simulink model "Estimations"  (R2023a)
settings: Solver=FixedStepAuto  StartTime=0.0  StopTime=150000  FixedStep=1  RelTol=1e-3
InitFcn:
  | load BatteryParameters.mat
values from neighbouring files (symbols this model uses):
  C1_LUT = [540 560 568 572 576 580 600 620 640 660 680 700 ... (105 elements, 21x5)]    [BatteryParameters.mat]
  Em_LUT = [3.147 3.292 3.392 3.477 3.518 3.561 3.602 3.638 3.677 3.719 3.763 3.799 ... (105 elements, 21x5)]    [BatteryParameters.mat]
  R1_LUT = [0.153117539 0.114898532 0.101253199 0.093222981 0.089962592 0.089117306 0.088090887 0.087366356 0.086883336 0.086038049 0.08477012 0.085313519 ... (105 elements, 21x5)]    [BatteryParameters.mat]
  SOC_LUT = [0 0.05 0.1 0.15 0.2 0.25 0.3 0.35 0.4 0.45 0.5 0.55 ... (21 elements, 21x1)]    [BatteryParameters.mat]
  Temperature_LUT = [263.15 273.15 298.15 318.15 333.15]    [BatteryParameters.mat]
  Ts = 1    [BatteryParameters.mat]
libraries: sharedTrackingLibrary x9
(part 1 of 2)
settings Model: Creator=The MathWorks, Inc.  LastModifiedBy=10661326
settings SolverCC: AlgebraicLoopSolver=TrustRegion
settings DataIOCC: ReturnWorkspaceOutputs=off
settings OptimizationCC: DefaultParameterBehavior=Inlined  EnhancedBackFolding=on  PassReuseOutputArgsAs=Individual arguments  ZeroExternalMemoryAtStartup=off  ZeroInternalMemoryAtStartup=off  OptimizeBlockOrder=speed  DifferentSizesBufferReuse=on  OptimizationCustomize=off  EfficientTunableParamExpr=on
settings DebuggingCC: ParameterTunabilityLossMsg=error  UnconnectedInputMsg=warning  UnconnectedOutputMsg=warning  UnconnectedLineMsg=warning  ArithmeticOperatorsInVariantConditions=warning
settings HardwareCC: ProdBitPerChar=16  ProdBitPerInt=16  ProdBitPerPointer=32  ProdBitPerSizeT=32  ProdBitPerPtrDiffT=32  ProdLargestAtomicInteger=Integer  ProdLargestAtomicFloat=None  ProdWordSize=16  ProdHWDeviceType=Texas Instruments->C2000
settings ModelReferenceCC: EnableRefExpFcnMdlSchedulingChecks=on
settings SFSimCC: SimUseLocalCustomCode=off  MATLABDynamicMemAlloc=off  CustomCodeUndefinedFunction=UseInterfaceOnly
settings RTWCC: Description=Embedded Coder  SystemTargetFile=ert.tlc  TemplateMakefile=ert_default_tmf  RTWUseLocalCustomCode=off  DLArmComputeVersion=19.05
settings CodeAppCC: ForceParamTrailComments=on  IgnoreCustomStorageClasses=off  OperatorAnnotations=on  SimulinkDataObjDesc=on  SFDataObjDesc=on  InsertBlockDesc=on
settings ERTTargetCC: TargetLangStandard=C99 (ISO)  GenerateSampleERTMain=on  InlinedParameterPlacement=NonHierarchical  ERTCustomFileTemplate=example_file_process.tlc
settings SimscapeCC: SimscapeNormalizeSystem=off

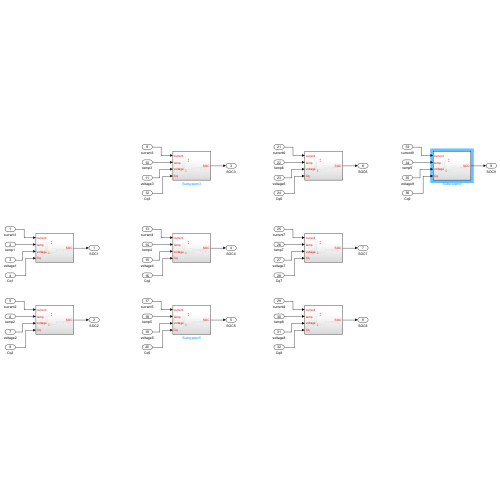
[thumbnail: Simulink's stored preview of the top-level diagram]
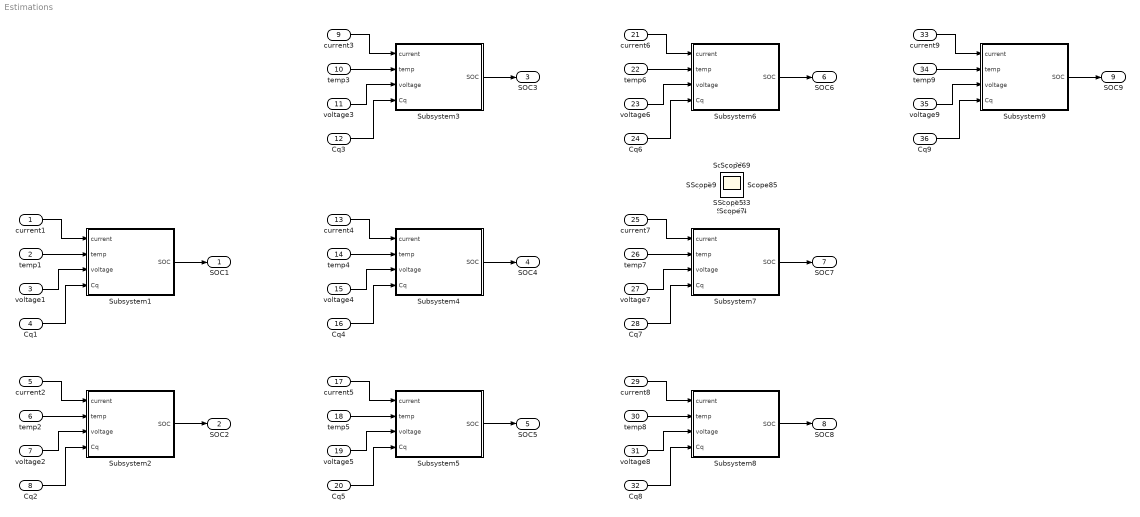
== system Estimations ==
  current1 : Inport
  temp1 : Inport  Port=2
  voltage1 : Inport  Port=3
  Cq1 : Inport  Port=4
  current2 : Inport  Port=5
  temp2 : Inport  Port=6
  voltage2 : Inport  Port=7
  Cq2 : Inport  Port=8
  current3 : Inport  Port=9
  temp3 : Inport  Port=10
  voltage3 : Inport  Port=11
  Cq3 : Inport  Port=12
  current4 : Inport  Port=13
  temp4 : Inport  Port=14
  voltage4 : Inport  Port=15
  Cq4 : Inport  Port=16
  current5 : Inport  Port=17
  temp5 : Inport  Port=18
  voltage5 : Inport  Port=19
  Cq5 : Inport  Port=20
  current6 : Inport  Port=21
  temp6 : Inport  Port=22
  voltage6 : Inport  Port=23
  Cq6 : Inport  Port=24
  current7 : Inport  Port=25
  temp7 : Inport  Port=26
  voltage7 : Inport  Port=27
  Cq7 : Inport  Port=28
  current8 : Inport  Port=29
  temp8 : Inport  Port=30
  voltage8 : Inport  Port=31
  Cq8 : Inport  Port=32
  current9 : Inport  Port=33
  temp9 : Inport  Port=34
  voltage9 : Inport  Port=35
  Cq9 : Inport  Port=36
  Subsystem1 : Subsystem
  Subsystem2 : Subsystem
  Subsystem3 : Subsystem
  Subsystem4 : Subsystem
  Subsystem5 : Subsystem
  Subsystem6 : Subsystem
  Subsystem7 : Subsystem
  Subsystem8 : Subsystem
  Subsystem9 : Subsystem
  SOC1 : Outport
  SOC2 : Outport  Port=2
  SOC3 : Outport  Port=3
  SOC4 : Outport  Port=4
  SOC5 : Outport  Port=5
  SOC6 : Outport  Port=6
  SOC7 : Outport  Port=7
  SOC8 : Outport  Port=8
  SOC9 : Outport  Port=9
  Scope{,1..11,13,17..18,20,22..35} (30 alike) : Scope
  wires:
  Subsystem1/1(SOC) -> SOC1/1
  Cq1/1 -> Subsystem1/4(Cq)
  current1/1 -> Subsystem1/1(current)
  temp1/1 -> Subsystem1/2(temp)
  voltage1/1 -> Subsystem1/3(voltage)
  voltage2/1 -> Subsystem2/3(voltage)
  temp2/1 -> Subsystem2/2(temp)
  current2/1 -> Subsystem2/1(current)
  Cq2/1 -> Subsystem2/4(Cq)
  Subsystem2/1(SOC) -> SOC2/1
  Subsystem5/1(SOC) -> SOC5/1
  Cq5/1 -> Subsystem5/4(Cq)
  current5/1 -> Subsystem5/1(current)
  temp5/1 -> Subsystem5/2(temp)
  voltage5/1 -> Subsystem5/3(voltage)
  voltage4/1 -> Subsystem4/3(voltage)
  temp4/1 -> Subsystem4/2(temp)
  current4/1 -> Subsystem4/1(current)
  Cq4/1 -> Subsystem4/4(Cq)
  Subsystem4/1(SOC) -> SOC4/1
  Subsystem3/1(SOC) -> SOC3/1
  Cq3/1 -> Subsystem3/4(Cq)
  current3/1 -> Subsystem3/1(current)
  temp3/1 -> Subsystem3/2(temp)
  voltage3/1 -> Subsystem3/3(voltage)
  voltage6/1 -> Subsystem6/3(voltage)
  temp6/1 -> Subsystem6/2(temp)
  current6/1 -> Subsystem6/1(current)
  Cq6/1 -> Subsystem6/4(Cq)
  Subsystem6/1(SOC) -> SOC6/1
  Subsystem7/1(SOC) -> SOC7/1
  Cq7/1 -> Subsystem7/4(Cq)
  current7/1 -> Subsystem7/1(current)
  temp7/1 -> Subsystem7/2(temp)
  voltage7/1 -> Subsystem7/3(voltage)
  voltage8/1 -> Subsystem8/3(voltage)
  temp8/1 -> Subsystem8/2(temp)
  current8/1 -> Subsystem8/1(current)
  Cq8/1 -> Subsystem8/4(Cq)
  Subsystem8/1(SOC) -> SOC8/1
  Subsystem9/1(SOC) -> SOC9/1
  Cq9/1 -> Subsystem9/4(Cq)
  current9/1 -> Subsystem9/1(current)
  temp9/1 -> Subsystem9/2(temp)
  voltage9/1 -> Subsystem9/3(voltage)

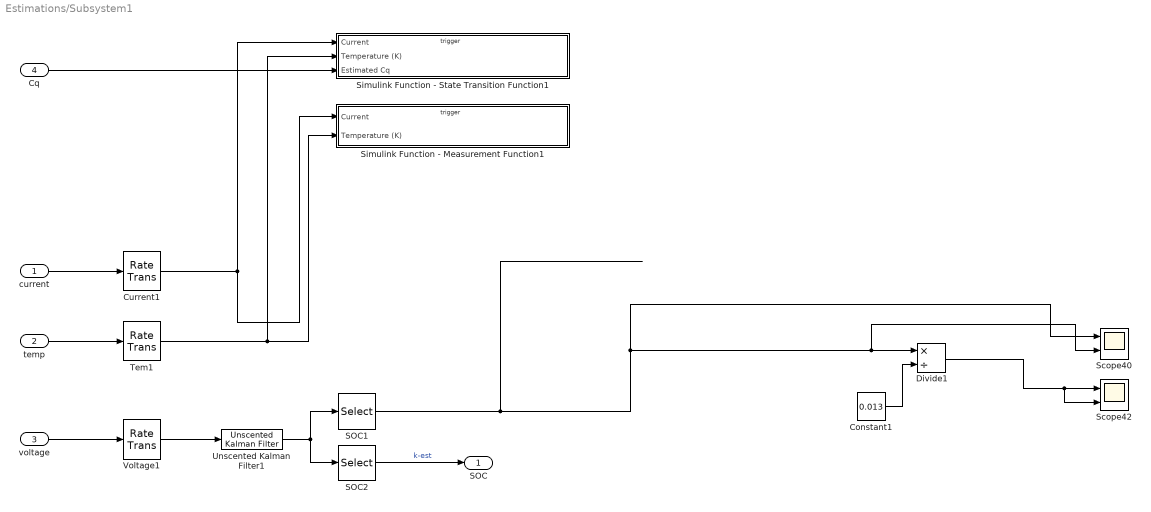
== system Estimations/Subsystem1 ==
  current : Inport
  temp : Inport  Port=2
  voltage : Inport  Port=3
  Cq : Inport  Port=4
  Constant1 : Constant  Value=0.013
  Current1 : RateTransition  OutPortSampleTime=Ts
  Divide1 : Product  Inputs=*/
  SOC1 : Selector  InputPortWidth=3  IndexOptions=Index vector (dialog)  Indices=3  OutputSizes=1
  SOC2 : Selector  InputPortWidth=3  IndexOptions=Index vector (dialog)  Indices=1  OutputSizes=1
  Scope40 : Scope  NumInputPorts=2
  Scope42 : Scope  NumInputPorts=2
  Simulink Function - Measurement Function1 : Subsystem  TreatAsAtomicUnit=on
  Simulink Function - State Transition Function1 : Subsystem  TreatAsAtomicUnit=on
  Tem1 : RateTransition  InitialCondition=300  OutPortSampleTime=Ts
  Unscented Kalman Filter1 : sharedTrackingLibrary/Unscented Kalman Filter  StateTransitionFcn=batteryStateFcn1  HasAdditiveProcessNoise=Additive  ProcessNoise=diag([2e-8, 3e-7, 2e-8])  HasTimeVaryingProcessNoise=off  HasStateTransitionFcnExtraArgument=0  InitialState=[0.5; 0; 0.01]  InitialStateCovariance=diag([0.01, 1,1])  Alpha=1  Beta=2  Kappa=0  MeasurementFcn1=batteryMeasurementFcn1  HasMeasurementEnablePort1=off  HasAdditiveMeasurementNoise1=Additive  MeasurementNoise1=1e-3  HasTimeVaryingMeasurementNoise1=off  HasMeasurementFcnExtraArgument1=0  HasMeasurementWrapping1=off  MeasurementFcn2=myMeasurementFcn  HasMeasurementEnablePort2=off  HasAdditiveMeasurementNoise2=Additive  MeasurementNoise2=1  HasTimeVaryingMeasurementNoise2=off  HasMeasurementFcnExtraArgument2=0  HasMeasurementWrapping2=off  MeasurementFcn3=myMeasurementFcn  HasMeasurementEnablePort3=off  HasAdditiveMeasurementNoise3=Additive  MeasurementNoise3=1  HasTimeVaryingMeasurementNoise3=off  HasMeasurementFcnExtraArgument3=0  HasMeasurementWrapping3=off  MeasurementFcn4=myMeasurementFcn  HasMeasurementEnablePort4=off  HasAdditiveMeasurementNoise4=Additive  MeasurementNoise4=1  HasTimeVaryingMeasurementNoise4=off  HasMeasurementFcnExtraArgument4=0  HasMeasurementWrapping4=off  MeasurementFcn5=myMeasurementFcn  HasMeasurementEnablePort5=off  HasAdditiveMeasurementNoise5=Additive  MeasurementNoise5=1  HasTimeVaryingMeasurementNoise5=off  HasMeasurementFcnExtraArgument5=0  HasMeasurementWrapping5=off  EnableMultirate=off  StateTransitionFcnSampleTime=-1  MeasurementFcn1SampleTime=-1  MeasurementFcn2SampleTime=-1  MeasurementFcn3SampleTime=-1  MeasurementFcn4SampleTime=-1  MeasurementFcn5SampleTime=-1  UseCurrentEstimator=on  OutputStateCovariance=off  DataType=double  SampleTime=Ts  NumberOfMeasurements=1
  Voltage1 : RateTransition  InitialCondition=4  OutPortSampleTime=Ts
  SOC : Outport
  wires:
  Cq/1 -> Simulink Function - State Transition Function1/3(Estimated Cq)
  voltage/1 -> Voltage1/1
  Tem1/1 -> Simulink Function - Measurement Function1/2(Temperature (K)), Simulink Function - State Transition Function1/2(Temperature (K))
  Current1/1 -> Simulink Function - State Transition Function1/1(Current), Simulink Function - Measurement Function1/1(Current)
  current/1 -> Current1/1
  temp/1 -> Tem1/1
  Divide1/1 -> Scope42/1, Scope42/2
  Unscented Kalman Filter1/1 -> SOC2/1, SOC1/1
  SOC2/1 -> SOC/1  "k-est"
  Voltage1/1 -> Unscented Kalman Filter1/1
  Constant1/1 -> Divide1/2
  SOC1/1 -> Scope40/1, Divide1/1, Scope40/2

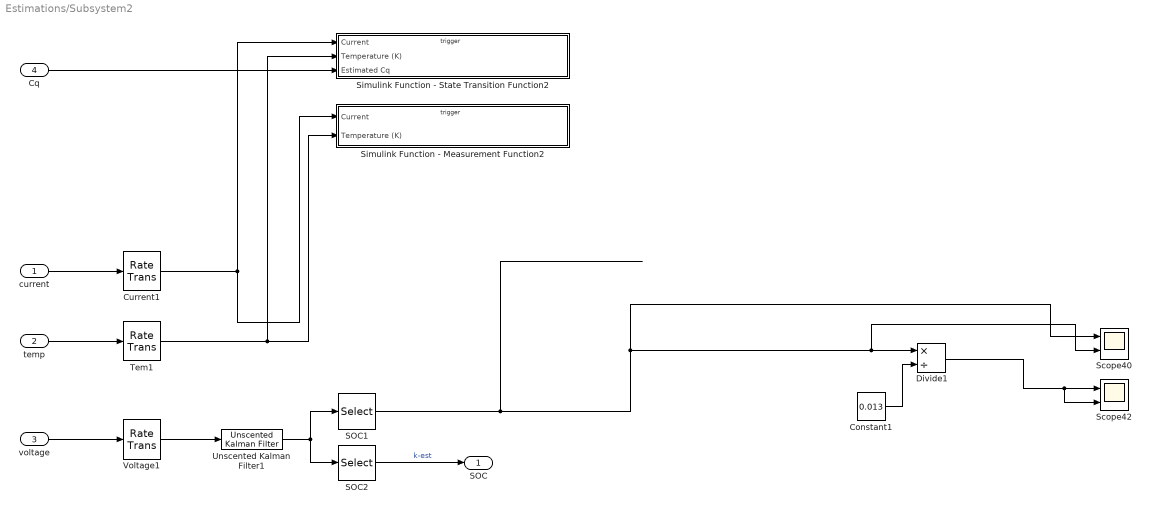
== system Estimations/Subsystem2 ==
  current : Inport
  temp : Inport  Port=2
  voltage : Inport  Port=3
  Cq : Inport  Port=4
  Constant1 : Constant  Value=0.013
  Current1 : RateTransition  OutPortSampleTime=Ts
  Divide1 : Product  Inputs=*/
  SOC1 : Selector  InputPortWidth=3  IndexOptions=Index vector (dialog)  Indices=3  OutputSizes=1
  SOC2 : Selector  InputPortWidth=3  IndexOptions=Index vector (dialog)  Indices=1  OutputSizes=1
  Scope40 : Scope  NumInputPorts=2
  Scope42 : Scope  NumInputPorts=2
  Simulink Function - Measurement Function2 : Subsystem  TreatAsAtomicUnit=on
  Simulink Function - State Transition Function2 : Subsystem  TreatAsAtomicUnit=on
  Tem1 : RateTransition  InitialCondition=300  OutPortSampleTime=Ts
  Unscented Kalman Filter1 : sharedTrackingLibrary/Unscented Kalman Filter  StateTransitionFcn=batteryStateFcn2  HasAdditiveProcessNoise=Additive  ProcessNoise=diag([2e-8, 3e-7, 2e-8])  HasTimeVaryingProcessNoise=off  HasStateTransitionFcnExtraArgument=0  InitialState=[0.5; 0; 0.01]  InitialStateCovariance=diag([0.01, 1,1])  Alpha=1  Beta=2  Kappa=0  MeasurementFcn1=batteryMeasurementFcn2  HasMeasurementEnablePort1=off  HasAdditiveMeasurementNoise1=Additive  MeasurementNoise1=1e-3  HasTimeVaryingMeasurementNoise1=off  HasMeasurementFcnExtraArgument1=0  HasMeasurementWrapping1=off  MeasurementFcn2=myMeasurementFcn  HasMeasurementEnablePort2=off  HasAdditiveMeasurementNoise2=Additive  MeasurementNoise2=1  HasTimeVaryingMeasurementNoise2=off  HasMeasurementFcnExtraArgument2=0  HasMeasurementWrapping2=off  MeasurementFcn3=myMeasurementFcn  HasMeasurementEnablePort3=off  HasAdditiveMeasurementNoise3=Additive  MeasurementNoise3=1  HasTimeVaryingMeasurementNoise3=off  HasMeasurementFcnExtraArgument3=0  HasMeasurementWrapping3=off  MeasurementFcn4=myMeasurementFcn  HasMeasurementEnablePort4=off  HasAdditiveMeasurementNoise4=Additive  MeasurementNoise4=1  HasTimeVaryingMeasurementNoise4=off  HasMeasurementFcnExtraArgument4=0  HasMeasurementWrapping4=off  MeasurementFcn5=myMeasurementFcn  HasMeasurementEnablePort5=off  HasAdditiveMeasurementNoise5=Additive  MeasurementNoise5=1  HasTimeVaryingMeasurementNoise5=off  HasMeasurementFcnExtraArgument5=0  HasMeasurementWrapping5=off  EnableMultirate=off  StateTransitionFcnSampleTime=-1  MeasurementFcn1SampleTime=-1  MeasurementFcn2SampleTime=-1  MeasurementFcn3SampleTime=-1  MeasurementFcn4SampleTime=-1  MeasurementFcn5SampleTime=-1  UseCurrentEstimator=on  OutputStateCovariance=off  DataType=double  SampleTime=Ts  NumberOfMeasurements=1
  Voltage1 : RateTransition  InitialCondition=4  OutPortSampleTime=Ts
  SOC : Outport
  wires:
  SOC1/1 -> Scope40/2, Divide1/1, Scope40/1
  Constant1/1 -> Divide1/2
  Voltage1/1 -> Unscented Kalman Filter1/1
  SOC2/1 -> SOC/1  "k-est"
  Unscented Kalman Filter1/1 -> SOC1/1, SOC2/1
  Divide1/1 -> Scope42/2, Scope42/1
  temp/1 -> Tem1/1
  current/1 -> Current1/1
  Current1/1 -> Simulink Function - Measurement Function2/1(Current), Simulink Function - State Transition Function2/1(Current)
  Tem1/1 -> Simulink Function - State Transition Function2/2(Temperature (K)), Simulink Function - Measurement Function2/2(Temperature (K))
  voltage/1 -> Voltage1/1
  Cq/1 -> Simulink Function - State Transition Function2/3(Estimated Cq)

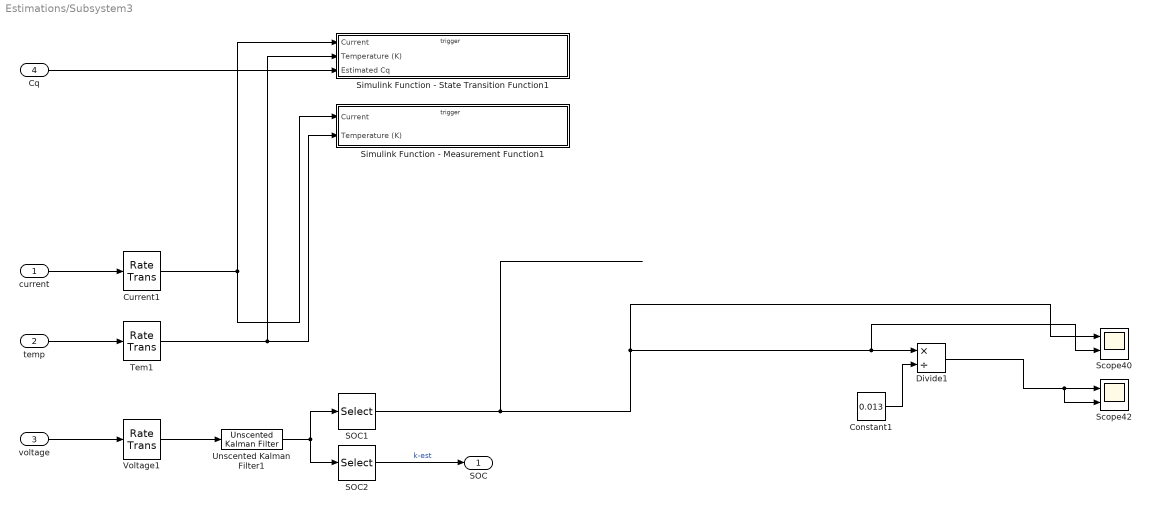
== system Estimations/Subsystem3 ==
  current : Inport
  temp : Inport  Port=2
  voltage : Inport  Port=3
  Cq : Inport  Port=4
  Constant1 : Constant  Value=0.013
  Current1 : RateTransition  OutPortSampleTime=Ts
  Divide1 : Product  Inputs=*/
  SOC1 : Selector  InputPortWidth=3  IndexOptions=Index vector (dialog)  Indices=3  OutputSizes=1
  SOC2 : Selector  InputPortWidth=3  IndexOptions=Index vector (dialog)  Indices=1  OutputSizes=1
  Scope40 : Scope  NumInputPorts=2
  Scope42 : Scope  NumInputPorts=2
  Simulink Function - Measurement Function1 : Subsystem  TreatAsAtomicUnit=on
  Simulink Function - State Transition Function1 : Subsystem  TreatAsAtomicUnit=on
  Tem1 : RateTransition  InitialCondition=300  OutPortSampleTime=Ts
  Unscented Kalman Filter1 : sharedTrackingLibrary/Unscented Kalman Filter  StateTransitionFcn=batteryStateFcn3  HasAdditiveProcessNoise=Additive  ProcessNoise=diag([2e-8, 3e-7, 2e-8])  HasTimeVaryingProcessNoise=off  HasStateTransitionFcnExtraArgument=0  InitialState=[0.5; 0; 0.01]  InitialStateCovariance=diag([0.01, 1,1])  Alpha=1  Beta=2  Kappa=0  MeasurementFcn1=batteryMeasurementFcn3  HasMeasurementEnablePort1=off  HasAdditiveMeasurementNoise1=Additive  MeasurementNoise1=1e-3  HasTimeVaryingMeasurementNoise1=off  HasMeasurementFcnExtraArgument1=0  HasMeasurementWrapping1=off  MeasurementFcn2=myMeasurementFcn  HasMeasurementEnablePort2=off  HasAdditiveMeasurementNoise2=Additive  MeasurementNoise2=1  HasTimeVaryingMeasurementNoise2=off  HasMeasurementFcnExtraArgument2=0  HasMeasurementWrapping2=off  MeasurementFcn3=myMeasurementFcn  HasMeasurementEnablePort3=off  HasAdditiveMeasurementNoise3=Additive  MeasurementNoise3=1  HasTimeVaryingMeasurementNoise3=off  HasMeasurementFcnExtraArgument3=0  HasMeasurementWrapping3=off  MeasurementFcn4=myMeasurementFcn  HasMeasurementEnablePort4=off  HasAdditiveMeasurementNoise4=Additive  MeasurementNoise4=1  HasTimeVaryingMeasurementNoise4=off  HasMeasurementFcnExtraArgument4=0  HasMeasurementWrapping4=off  MeasurementFcn5=myMeasurementFcn  HasMeasurementEnablePort5=off  HasAdditiveMeasurementNoise5=Additive  MeasurementNoise5=1  HasTimeVaryingMeasurementNoise5=off  HasMeasurementFcnExtraArgument5=0  HasMeasurementWrapping5=off  EnableMultirate=off  StateTransitionFcnSampleTime=-1  MeasurementFcn1SampleTime=-1  MeasurementFcn2SampleTime=-1  MeasurementFcn3SampleTime=-1  MeasurementFcn4SampleTime=-1  MeasurementFcn5SampleTime=-1  UseCurrentEstimator=on  OutputStateCovariance=off  DataType=double  SampleTime=Ts  NumberOfMeasurements=1
  Voltage1 : RateTransition  InitialCondition=4  OutPortSampleTime=Ts
  SOC : Outport
  wires:
  Cq/1 -> Simulink Function - State Transition Function1/3(Estimated Cq)
  voltage/1 -> Voltage1/1
  Tem1/1 -> Simulink Function - Measurement Function1/2(Temperature (K)), Simulink Function - State Transition Function1/2(Temperature (K))
  Current1/1 -> Simulink Function - State Transition Function1/1(Current), Simulink Function - Measurement Function1/1(Current)
  current/1 -> Current1/1
  temp/1 -> Tem1/1
  Divide1/1 -> Scope42/1, Scope42/2
  Unscented Kalman Filter1/1 -> SOC2/1, SOC1/1
  SOC2/1 -> SOC/1  "k-est"
  Voltage1/1 -> Unscented Kalman Filter1/1
  Constant1/1 -> Divide1/2
  SOC1/1 -> Scope40/1, Divide1/1, Scope40/2

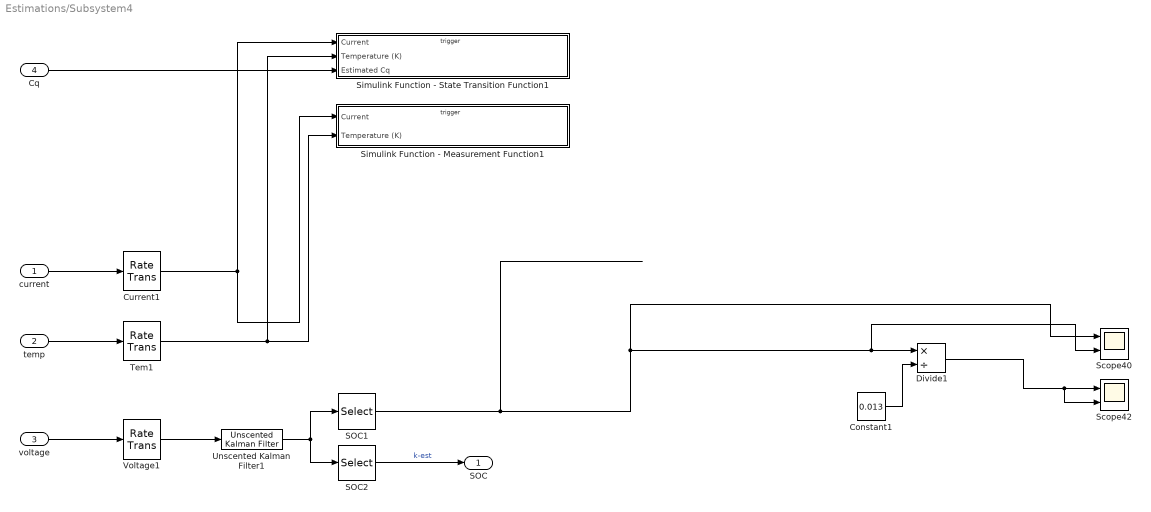
== system Estimations/Subsystem4 ==
  current : Inport
  temp : Inport  Port=2
  voltage : Inport  Port=3
  Cq : Inport  Port=4
  Constant1 : Constant  Value=0.013
  Current1 : RateTransition  OutPortSampleTime=Ts
  Divide1 : Product  Inputs=*/
  SOC1 : Selector  InputPortWidth=3  IndexOptions=Index vector (dialog)  Indices=3  OutputSizes=1
  SOC2 : Selector  InputPortWidth=3  IndexOptions=Index vector (dialog)  Indices=1  OutputSizes=1
  Scope40 : Scope  NumInputPorts=2
  Scope42 : Scope  NumInputPorts=2
  Simulink Function - Measurement Function1 : Subsystem  TreatAsAtomicUnit=on
  Simulink Function - State Transition Function1 : Subsystem  TreatAsAtomicUnit=on
  Tem1 : RateTransition  InitialCondition=300  OutPortSampleTime=Ts
  Unscented Kalman Filter1 : sharedTrackingLibrary/Unscented Kalman Filter  StateTransitionFcn=batteryStateFcn4  HasAdditiveProcessNoise=Additive  ProcessNoise=diag([2e-8, 3e-7, 2e-8])  HasTimeVaryingProcessNoise=off  HasStateTransitionFcnExtraArgument=0  InitialState=[0.5; 0; 0.01]  InitialStateCovariance=diag([0.01, 1,1])  Alpha=1  Beta=2  Kappa=0  MeasurementFcn1=batteryMeasurementFcn4  HasMeasurementEnablePort1=off  HasAdditiveMeasurementNoise1=Additive  MeasurementNoise1=1e-3  HasTimeVaryingMeasurementNoise1=off  HasMeasurementFcnExtraArgument1=0  HasMeasurementWrapping1=off  MeasurementFcn2=myMeasurementFcn  HasMeasurementEnablePort2=off  HasAdditiveMeasurementNoise2=Additive  MeasurementNoise2=1  HasTimeVaryingMeasurementNoise2=off  HasMeasurementFcnExtraArgument2=0  HasMeasurementWrapping2=off  MeasurementFcn3=myMeasurementFcn  HasMeasurementEnablePort3=off  HasAdditiveMeasurementNoise3=Additive  MeasurementNoise3=1  HasTimeVaryingMeasurementNoise3=off  HasMeasurementFcnExtraArgument3=0  HasMeasurementWrapping3=off  MeasurementFcn4=myMeasurementFcn  HasMeasurementEnablePort4=off  HasAdditiveMeasurementNoise4=Additive  MeasurementNoise4=1  HasTimeVaryingMeasurementNoise4=off  HasMeasurementFcnExtraArgument4=0  HasMeasurementWrapping4=off  MeasurementFcn5=myMeasurementFcn  HasMeasurementEnablePort5=off  HasAdditiveMeasurementNoise5=Additive  MeasurementNoise5=1  HasTimeVaryingMeasurementNoise5=off  HasMeasurementFcnExtraArgument5=0  HasMeasurementWrapping5=off  EnableMultirate=off  StateTransitionFcnSampleTime=-1  MeasurementFcn1SampleTime=-1  MeasurementFcn2SampleTime=-1  MeasurementFcn3SampleTime=-1  MeasurementFcn4SampleTime=-1  MeasurementFcn5SampleTime=-1  UseCurrentEstimator=on  OutputStateCovariance=off  DataType=double  SampleTime=Ts  NumberOfMeasurements=1
  Voltage1 : RateTransition  InitialCondition=4  OutPortSampleTime=Ts
  SOC : Outport
  wires:
  SOC1/1 -> Scope40/2, Divide1/1, Scope40/1
  Constant1/1 -> Divide1/2
  Voltage1/1 -> Unscented Kalman Filter1/1
  SOC2/1 -> SOC/1  "k-est"
  Unscented Kalman Filter1/1 -> SOC1/1, SOC2/1
  Divide1/1 -> Scope42/2, Scope42/1
  temp/1 -> Tem1/1
  current/1 -> Current1/1
  Current1/1 -> Simulink Function - Measurement Function1/1(Current), Simulink Function - State Transition Function1/1(Current)
  Tem1/1 -> Simulink Function - State Transition Function1/2(Temperature (K)), Simulink Function - Measurement Function1/2(Temperature (K))
  voltage/1 -> Voltage1/1
  Cq/1 -> Simulink Function - State Transition Function1/3(Estimated Cq)

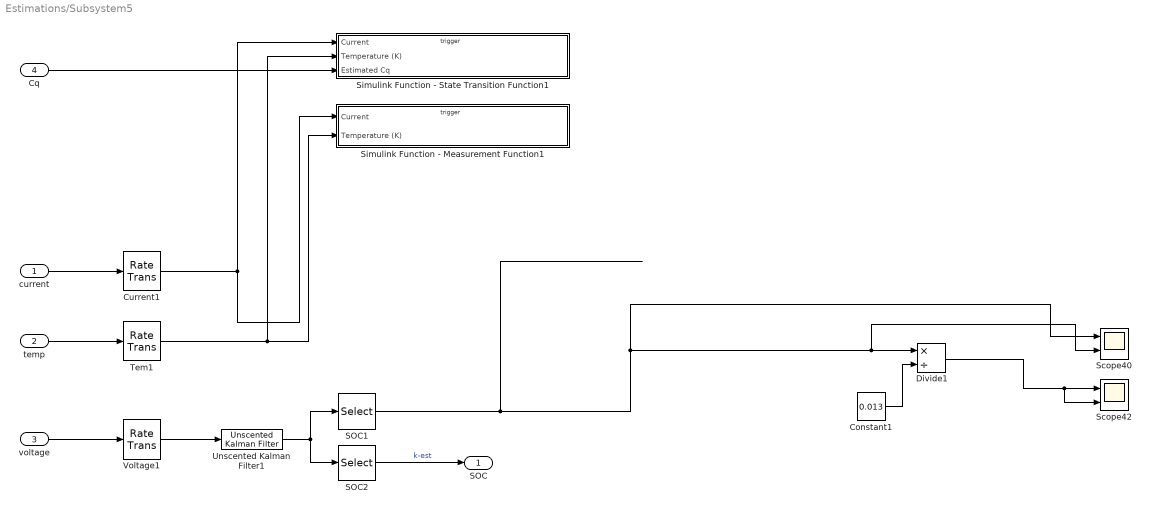
== system Estimations/Subsystem5 ==
  current : Inport
  temp : Inport  Port=2
  voltage : Inport  Port=3
  Cq : Inport  Port=4
  Constant1 : Constant  Value=0.013
  Current1 : RateTransition  OutPortSampleTime=Ts
  Divide1 : Product  Inputs=*/
  SOC1 : Selector  InputPortWidth=3  IndexOptions=Index vector (dialog)  Indices=3  OutputSizes=1
  SOC2 : Selector  InputPortWidth=3  IndexOptions=Index vector (dialog)  Indices=1  OutputSizes=1
  Scope40 : Scope  NumInputPorts=2
  Scope42 : Scope  NumInputPorts=2
  Simulink Function - Measurement Function1 : Subsystem  TreatAsAtomicUnit=on
  Simulink Function - State Transition Function1 : Subsystem  TreatAsAtomicUnit=on
  Tem1 : RateTransition  InitialCondition=300  OutPortSampleTime=Ts
  Unscented Kalman Filter1 : sharedTrackingLibrary/Unscented Kalman Filter  StateTransitionFcn=batteryStateFcn5  HasAdditiveProcessNoise=Additive  ProcessNoise=diag([2e-8, 3e-7, 2e-8])  HasTimeVaryingProcessNoise=off  HasStateTransitionFcnExtraArgument=0  InitialState=[0.5; 0; 0.01]  InitialStateCovariance=diag([0.01, 1,1])  Alpha=1  Beta=2  Kappa=0  MeasurementFcn1=batteryMeasurementFcn5  HasMeasurementEnablePort1=off  HasAdditiveMeasurementNoise1=Additive  MeasurementNoise1=1e-3  HasTimeVaryingMeasurementNoise1=off  HasMeasurementFcnExtraArgument1=0  HasMeasurementWrapping1=off  MeasurementFcn2=myMeasurementFcn  HasMeasurementEnablePort2=off  HasAdditiveMeasurementNoise2=Additive  MeasurementNoise2=1  HasTimeVaryingMeasurementNoise2=off  HasMeasurementFcnExtraArgument2=0  HasMeasurementWrapping2=off  MeasurementFcn3=myMeasurementFcn  HasMeasurementEnablePort3=off  HasAdditiveMeasurementNoise3=Additive  MeasurementNoise3=1  HasTimeVaryingMeasurementNoise3=off  HasMeasurementFcnExtraArgument3=0  HasMeasurementWrapping3=off  MeasurementFcn4=myMeasurementFcn  HasMeasurementEnablePort4=off  HasAdditiveMeasurementNoise4=Additive  MeasurementNoise4=1  HasTimeVaryingMeasurementNoise4=off  HasMeasurementFcnExtraArgument4=0  HasMeasurementWrapping4=off  MeasurementFcn5=myMeasurementFcn  HasMeasurementEnablePort5=off  HasAdditiveMeasurementNoise5=Additive  MeasurementNoise5=1  HasTimeVaryingMeasurementNoise5=off  HasMeasurementFcnExtraArgument5=0  HasMeasurementWrapping5=off  EnableMultirate=off  StateTransitionFcnSampleTime=-1  MeasurementFcn1SampleTime=-1  MeasurementFcn2SampleTime=-1  MeasurementFcn3SampleTime=-1  MeasurementFcn4SampleTime=-1  MeasurementFcn5SampleTime=-1  UseCurrentEstimator=on  OutputStateCovariance=off  DataType=double  SampleTime=Ts  NumberOfMeasurements=1
  Voltage1 : RateTransition  InitialCondition=4  OutPortSampleTime=Ts
  SOC : Outport
  wires:
  Cq/1 -> Simulink Function - State Transition Function1/3(Estimated Cq)
  voltage/1 -> Voltage1/1
  Tem1/1 -> Simulink Function - Measurement Function1/2(Temperature (K)), Simulink Function - State Transition Function1/2(Temperature (K))
  Current1/1 -> Simulink Function - State Transition Function1/1(Current), Simulink Function - Measurement Function1/1(Current)
  current/1 -> Current1/1
  temp/1 -> Tem1/1
  Divide1/1 -> Scope42/1, Scope42/2
  Unscented Kalman Filter1/1 -> SOC2/1, SOC1/1
  SOC2/1 -> SOC/1  "k-est"
  Voltage1/1 -> Unscented Kalman Filter1/1
  Constant1/1 -> Divide1/2
  SOC1/1 -> Scope40/1, Divide1/1, Scope40/2

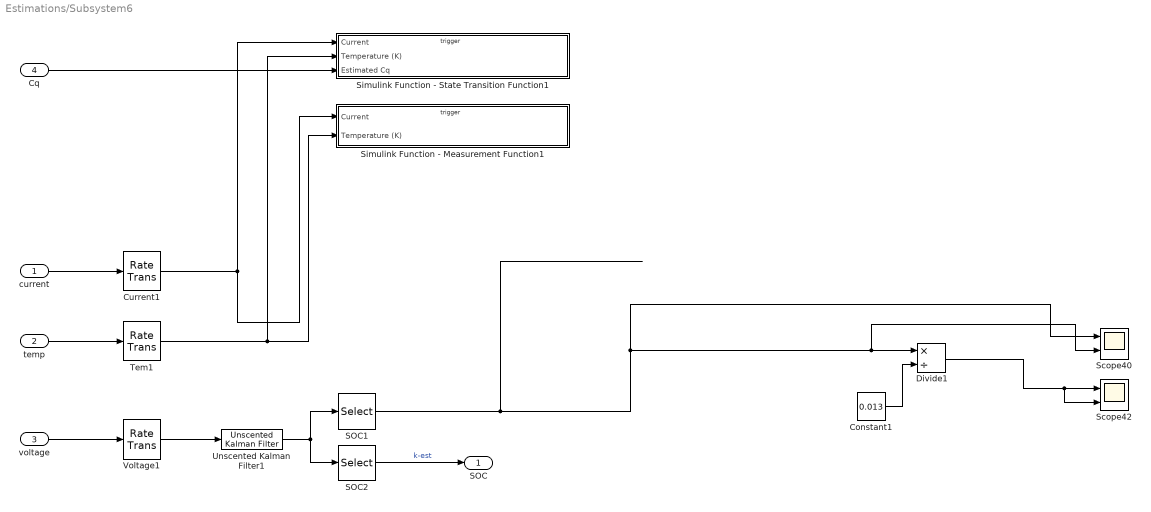
== system Estimations/Subsystem6 ==
  current : Inport
  temp : Inport  Port=2
  voltage : Inport  Port=3
  Cq : Inport  Port=4
  Constant1 : Constant  Value=0.013
  Current1 : RateTransition  OutPortSampleTime=Ts
  Divide1 : Product  Inputs=*/
  SOC1 : Selector  InputPortWidth=3  IndexOptions=Index vector (dialog)  Indices=3  OutputSizes=1
  SOC2 : Selector  InputPortWidth=3  IndexOptions=Index vector (dialog)  Indices=1  OutputSizes=1
  Scope40 : Scope  NumInputPorts=2
  Scope42 : Scope  NumInputPorts=2
  Simulink Function - Measurement Function1 : Subsystem  TreatAsAtomicUnit=on
  Simulink Function - State Transition Function1 : Subsystem  TreatAsAtomicUnit=on
  Tem1 : RateTransition  InitialCondition=300  OutPortSampleTime=Ts
  Unscented Kalman Filter1 : sharedTrackingLibrary/Unscented Kalman Filter  StateTransitionFcn=batteryStateFcn6  HasAdditiveProcessNoise=Additive  ProcessNoise=diag([2e-8, 3e-7, 2e-8])  HasTimeVaryingProcessNoise=off  HasStateTransitionFcnExtraArgument=0  InitialState=[0.5; 0; 0.01]  InitialStateCovariance=diag([0.01, 1,1])  Alpha=1  Beta=2  Kappa=0  MeasurementFcn1=batteryMeasurementFcn6  HasMeasurementEnablePort1=off  HasAdditiveMeasurementNoise1=Additive  MeasurementNoise1=1e-3  HasTimeVaryingMeasurementNoise1=off  HasMeasurementFcnExtraArgument1=0  HasMeasurementWrapping1=off  MeasurementFcn2=myMeasurementFcn  HasMeasurementEnablePort2=off  HasAdditiveMeasurementNoise2=Additive  MeasurementNoise2=1  HasTimeVaryingMeasurementNoise2=off  HasMeasurementFcnExtraArgument2=0  HasMeasurementWrapping2=off  MeasurementFcn3=myMeasurementFcn  HasMeasurementEnablePort3=off  HasAdditiveMeasurementNoise3=Additive  MeasurementNoise3=1  HasTimeVaryingMeasurementNoise3=off  HasMeasurementFcnExtraArgument3=0  HasMeasurementWrapping3=off  MeasurementFcn4=myMeasurementFcn  HasMeasurementEnablePort4=off  HasAdditiveMeasurementNoise4=Additive  MeasurementNoise4=1  HasTimeVaryingMeasurementNoise4=off  HasMeasurementFcnExtraArgument4=0  HasMeasurementWrapping4=off  MeasurementFcn5=myMeasurementFcn  HasMeasurementEnablePort5=off  HasAdditiveMeasurementNoise5=Additive  MeasurementNoise5=1  HasTimeVaryingMeasurementNoise5=off  HasMeasurementFcnExtraArgument5=0  HasMeasurementWrapping5=off  EnableMultirate=off  StateTransitionFcnSampleTime=-1  MeasurementFcn1SampleTime=-1  MeasurementFcn2SampleTime=-1  MeasurementFcn3SampleTime=-1  MeasurementFcn4SampleTime=-1  MeasurementFcn5SampleTime=-1  UseCurrentEstimator=on  OutputStateCovariance=off  DataType=double  SampleTime=Ts  NumberOfMeasurements=1
  Voltage1 : RateTransition  InitialCondition=4  OutPortSampleTime=Ts
  SOC : Outport
  wires:
  SOC1/1 -> Scope40/2, Divide1/1, Scope40/1
  Constant1/1 -> Divide1/2
  Voltage1/1 -> Unscented Kalman Filter1/1
  SOC2/1 -> SOC/1  "k-est"
  Unscented Kalman Filter1/1 -> SOC1/1, SOC2/1
  Divide1/1 -> Scope42/2, Scope42/1
  temp/1 -> Tem1/1
  current/1 -> Current1/1
  Current1/1 -> Simulink Function - Measurement Function1/1(Current), Simulink Function - State Transition Function1/1(Current)
  Tem1/1 -> Simulink Function - State Transition Function1/2(Temperature (K)), Simulink Function - Measurement Function1/2(Temperature (K))
  voltage/1 -> Voltage1/1
  Cq/1 -> Simulink Function - State Transition Function1/3(Estimated Cq)

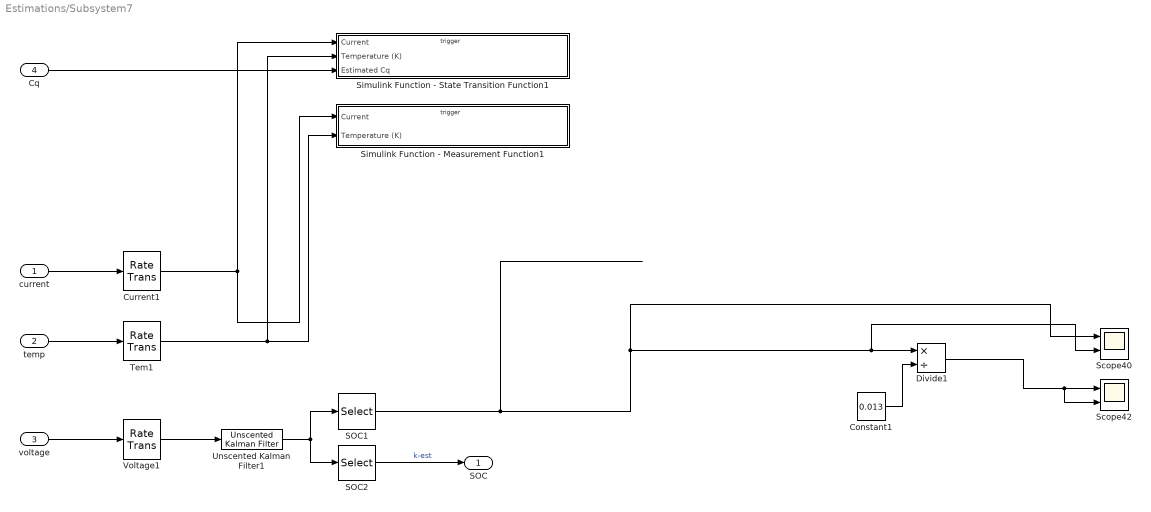
== system Estimations/Subsystem7 ==
  current : Inport
  temp : Inport  Port=2
  voltage : Inport  Port=3
  Cq : Inport  Port=4
  Constant1 : Constant  Value=0.013
  Current1 : RateTransition  OutPortSampleTime=Ts
  Divide1 : Product  Inputs=*/
  SOC1 : Selector  InputPortWidth=3  IndexOptions=Index vector (dialog)  Indices=3  OutputSizes=1
  SOC2 : Selector  InputPortWidth=3  IndexOptions=Index vector (dialog)  Indices=1  OutputSizes=1
  Scope40 : Scope  NumInputPorts=2
  Scope42 : Scope  NumInputPorts=2
  Simulink Function - Measurement Function1 : Subsystem  TreatAsAtomicUnit=on
  Simulink Function - State Transition Function1 : Subsystem  TreatAsAtomicUnit=on
  Tem1 : RateTransition  InitialCondition=300  OutPortSampleTime=Ts
  Unscented Kalman Filter1 : sharedTrackingLibrary/Unscented Kalman Filter  StateTransitionFcn=batteryStateFcn7  HasAdditiveProcessNoise=Additive  ProcessNoise=diag([2e-8, 3e-7, 2e-8])  HasTimeVaryingProcessNoise=off  HasStateTransitionFcnExtraArgument=0  InitialState=[0.5; 0; 0.01]  InitialStateCovariance=diag([0.01, 1,1])  Alpha=1  Beta=2  Kappa=0  MeasurementFcn1=batteryMeasurementFcn7  HasMeasurementEnablePort1=off  HasAdditiveMeasurementNoise1=Additive  MeasurementNoise1=1e-3  HasTimeVaryingMeasurementNoise1=off  HasMeasurementFcnExtraArgument1=0  HasMeasurementWrapping1=off  MeasurementFcn2=myMeasurementFcn  HasMeasurementEnablePort2=off  HasAdditiveMeasurementNoise2=Additive  MeasurementNoise2=1  HasTimeVaryingMeasurementNoise2=off  HasMeasurementFcnExtraArgument2=0  HasMeasurementWrapping2=off  MeasurementFcn3=myMeasurementFcn  HasMeasurementEnablePort3=off  HasAdditiveMeasurementNoise3=Additive  MeasurementNoise3=1  HasTimeVaryingMeasurementNoise3=off  HasMeasurementFcnExtraArgument3=0  HasMeasurementWrapping3=off  MeasurementFcn4=myMeasurementFcn  HasMeasurementEnablePort4=off  HasAdditiveMeasurementNoise4=Additive  MeasurementNoise4=1  HasTimeVaryingMeasurementNoise4=off  HasMeasurementFcnExtraArgument4=0  HasMeasurementWrapping4=off  MeasurementFcn5=myMeasurementFcn  HasMeasurementEnablePort5=off  HasAdditiveMeasurementNoise5=Additive  MeasurementNoise5=1  HasTimeVaryingMeasurementNoise5=off  HasMeasurementFcnExtraArgument5=0  HasMeasurementWrapping5=off  EnableMultirate=off  StateTransitionFcnSampleTime=-1  MeasurementFcn1SampleTime=-1  MeasurementFcn2SampleTime=-1  MeasurementFcn3SampleTime=-1  MeasurementFcn4SampleTime=-1  MeasurementFcn5SampleTime=-1  UseCurrentEstimator=on  OutputStateCovariance=off  DataType=double  SampleTime=Ts  NumberOfMeasurements=1
  Voltage1 : RateTransition  InitialCondition=4  OutPortSampleTime=Ts
  SOC : Outport
  wires:
  Cq/1 -> Simulink Function - State Transition Function1/3(Estimated Cq)
  voltage/1 -> Voltage1/1
  Tem1/1 -> Simulink Function - Measurement Function1/2(Temperature (K)), Simulink Function - State Transition Function1/2(Temperature (K))
  Current1/1 -> Simulink Function - State Transition Function1/1(Current), Simulink Function - Measurement Function1/1(Current)
  current/1 -> Current1/1
  temp/1 -> Tem1/1
  Divide1/1 -> Scope42/1, Scope42/2
  Unscented Kalman Filter1/1 -> SOC2/1, SOC1/1
  SOC2/1 -> SOC/1  "k-est"
  Voltage1/1 -> Unscented Kalman Filter1/1
  Constant1/1 -> Divide1/2
  SOC1/1 -> Scope40/1, Divide1/1, Scope40/2

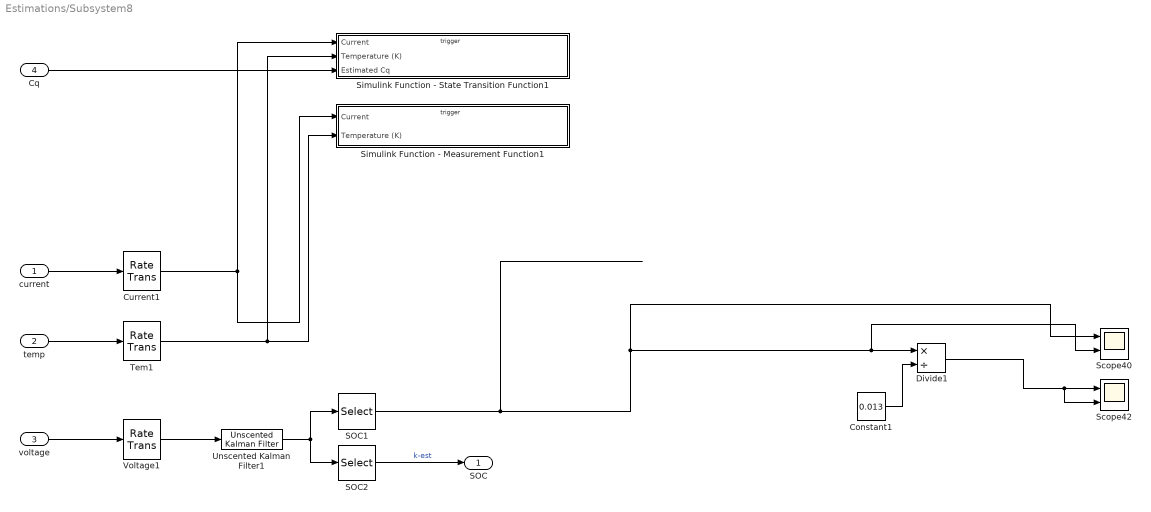
== system Estimations/Subsystem8 ==
  current : Inport
  temp : Inport  Port=2
  voltage : Inport  Port=3
  Cq : Inport  Port=4
  Constant1 : Constant  Value=0.013
  Current1 : RateTransition  OutPortSampleTime=Ts
  Divide1 : Product  Inputs=*/
  SOC1 : Selector  InputPortWidth=3  IndexOptions=Index vector (dialog)  Indices=3  OutputSizes=1
  SOC2 : Selector  InputPortWidth=3  IndexOptions=Index vector (dialog)  Indices=1  OutputSizes=1
  Scope40 : Scope  NumInputPorts=2
  Scope42 : Scope  NumInputPorts=2
  Simulink Function - Measurement Function1 : Subsystem  TreatAsAtomicUnit=on
  Simulink Function - State Transition Function1 : Subsystem  TreatAsAtomicUnit=on
  Tem1 : RateTransition  InitialCondition=300  OutPortSampleTime=Ts
  Unscented Kalman Filter1 : sharedTrackingLibrary/Unscented Kalman Filter  StateTransitionFcn=batteryStateFcn8  HasAdditiveProcessNoise=Additive  ProcessNoise=diag([2e-8, 3e-7, 2e-8])  HasTimeVaryingProcessNoise=off  HasStateTransitionFcnExtraArgument=0  InitialState=[0.5; 0; 0.01]  InitialStateCovariance=diag([0.01, 1,1])  Alpha=1  Beta=2  Kappa=0  MeasurementFcn1=batteryMeasurementFcn8  HasMeasurementEnablePort1=off  HasAdditiveMeasurementNoise1=Additive  MeasurementNoise1=1e-3  HasTimeVaryingMeasurementNoise1=off  HasMeasurementFcnExtraArgument1=0  HasMeasurementWrapping1=off  MeasurementFcn2=myMeasurementFcn  HasMeasurementEnablePort2=off  HasAdditiveMeasurementNoise2=Additive  MeasurementNoise2=1  HasTimeVaryingMeasurementNoise2=off  HasMeasurementFcnExtraArgument2=0  HasMeasurementWrapping2=off  MeasurementFcn3=myMeasurementFcn  HasMeasurementEnablePort3=off  HasAdditiveMeasurementNoise3=Additive  MeasurementNoise3=1  HasTimeVaryingMeasurementNoise3=off  HasMeasurementFcnExtraArgument3=0  HasMeasurementWrapping3=off  MeasurementFcn4=myMeasurementFcn  HasMeasurementEnablePort4=off  HasAdditiveMeasurementNoise4=Additive  MeasurementNoise4=1  HasTimeVaryingMeasurementNoise4=off  HasMeasurementFcnExtraArgument4=0  HasMeasurementWrapping4=off  MeasurementFcn5=myMeasurementFcn  HasMeasurementEnablePort5=off  HasAdditiveMeasurementNoise5=Additive  MeasurementNoise5=1  HasTimeVaryingMeasurementNoise5=off  HasMeasurementFcnExtraArgument5=0  HasMeasurementWrapping5=off  EnableMultirate=off  StateTransitionFcnSampleTime=-1  MeasurementFcn1SampleTime=-1  MeasurementFcn2SampleTime=-1  MeasurementFcn3SampleTime=-1  MeasurementFcn4SampleTime=-1  MeasurementFcn5SampleTime=-1  UseCurrentEstimator=on  OutputStateCovariance=off  DataType=double  SampleTime=Ts  NumberOfMeasurements=1
  Voltage1 : RateTransition  InitialCondition=4  OutPortSampleTime=Ts
  SOC : Outport
  wires:
  SOC1/1 -> Scope40/2, Divide1/1, Scope40/1
  Constant1/1 -> Divide1/2
  Voltage1/1 -> Unscented Kalman Filter1/1
  SOC2/1 -> SOC/1  "k-est"
  Unscented Kalman Filter1/1 -> SOC1/1, SOC2/1
  Divide1/1 -> Scope42/2, Scope42/1
  temp/1 -> Tem1/1
  current/1 -> Current1/1
  Current1/1 -> Simulink Function - Measurement Function1/1(Current), Simulink Function - State Transition Function1/1(Current)
  Tem1/1 -> Simulink Function - State Transition Function1/2(Temperature (K)), Simulink Function - Measurement Function1/2(Temperature (K))
  voltage/1 -> Voltage1/1
  Cq/1 -> Simulink Function - State Transition Function1/3(Estimated Cq)

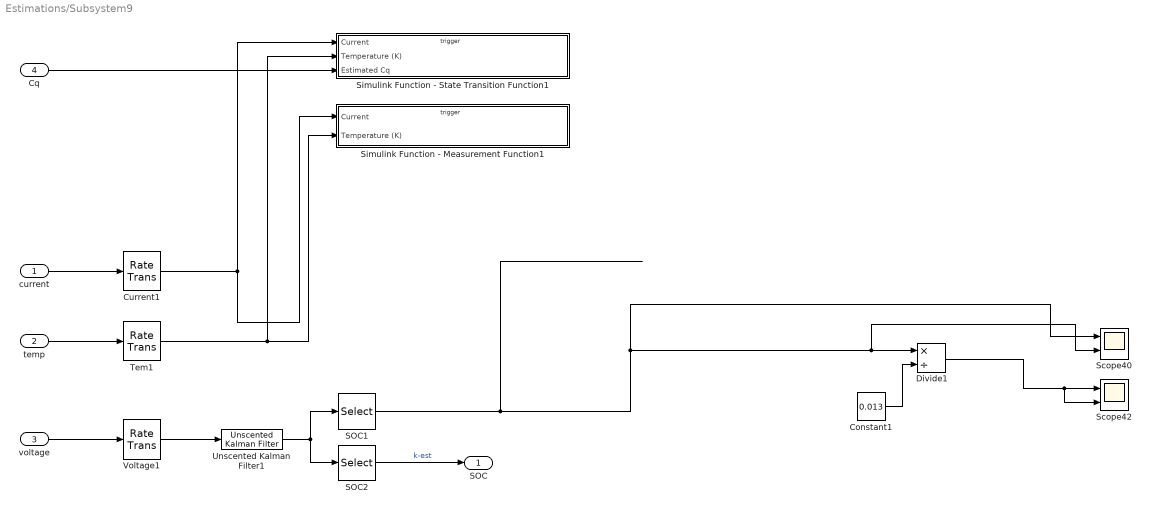
== system Estimations/Subsystem9 ==
  current : Inport
  temp : Inport  Port=2
  voltage : Inport  Port=3
  Cq : Inport  Port=4
  Constant1 : Constant  Value=0.013
  Current1 : RateTransition  OutPortSampleTime=Ts
  Divide1 : Product  Inputs=*/
  SOC1 : Selector  InputPortWidth=3  IndexOptions=Index vector (dialog)  Indices=3  OutputSizes=1
  SOC2 : Selector  InputPortWidth=3  IndexOptions=Index vector (dialog)  Indices=1  OutputSizes=1
  Scope40 : Scope  NumInputPorts=2
  Scope42 : Scope  NumInputPorts=2
  Simulink Function - Measurement Function1 : Subsystem  TreatAsAtomicUnit=on
  Simulink Function - State Transition Function1 : Subsystem  TreatAsAtomicUnit=on
  Tem1 : RateTransition  InitialCondition=300  OutPortSampleTime=Ts
  Unscented Kalman Filter1 : sharedTrackingLibrary/Unscented Kalman Filter  StateTransitionFcn=batteryStateFcn9  HasAdditiveProcessNoise=Additive  ProcessNoise=diag([2e-8, 3e-7, 2e-8])  HasTimeVaryingProcessNoise=off  HasStateTransitionFcnExtraArgument=0  InitialState=[0.5; 0; 0.01]  InitialStateCovariance=diag([0.01, 1,1])  Alpha=1  Beta=2  Kappa=0  MeasurementFcn1=batteryMeasurementFcn9  HasMeasurementEnablePort1=off  HasAdditiveMeasurementNoise1=Additive  MeasurementNoise1=1e-3  HasTimeVaryingMeasurementNoise1=off  HasMeasurementFcnExtraArgument1=0  HasMeasurementWrapping1=off  MeasurementFcn2=myMeasurementFcn  HasMeasurementEnablePort2=off  HasAdditiveMeasurementNoise2=Additive  MeasurementNoise2=1  HasTimeVaryingMeasurementNoise2=off  HasMeasurementFcnExtraArgument2=0  HasMeasurementWrapping2=off  MeasurementFcn3=myMeasurementFcn  HasMeasurementEnablePort3=off  HasAdditiveMeasurementNoise3=Additive  MeasurementNoise3=1  HasTimeVaryingMeasurementNoise3=off  HasMeasurementFcnExtraArgument3=0  HasMeasurementWrapping3=off  MeasurementFcn4=myMeasurementFcn  HasMeasurementEnablePort4=off  HasAdditiveMeasurementNoise4=Additive  MeasurementNoise4=1  HasTimeVaryingMeasurementNoise4=off  HasMeasurementFcnExtraArgument4=0  HasMeasurementWrapping4=off  MeasurementFcn5=myMeasurementFcn  HasMeasurementEnablePort5=off  HasAdditiveMeasurementNoise5=Additive  MeasurementNoise5=1  HasTimeVaryingMeasurementNoise5=off  HasMeasurementFcnExtraArgument5=0  HasMeasurementWrapping5=off  EnableMultirate=off  StateTransitionFcnSampleTime=-1  MeasurementFcn1SampleTime=-1  MeasurementFcn2SampleTime=-1  MeasurementFcn3SampleTime=-1  MeasurementFcn4SampleTime=-1  MeasurementFcn5SampleTime=-1  UseCurrentEstimator=on  OutputStateCovariance=off  DataType=double  SampleTime=Ts  NumberOfMeasurements=1
  Voltage1 : RateTransition  InitialCondition=4  OutPortSampleTime=Ts
  SOC : Outport
  wires:
  Cq/1 -> Simulink Function - State Transition Function1/3(Estimated Cq)
  voltage/1 -> Voltage1/1
  Tem1/1 -> Simulink Function - Measurement Function1/2(Temperature (K)), Simulink Function - State Transition Function1/2(Temperature (K))
  Current1/1 -> Simulink Function - State Transition Function1/1(Current), Simulink Function - Measurement Function1/1(Current)
  current/1 -> Current1/1
  temp/1 -> Tem1/1
  Divide1/1 -> Scope42/1, Scope42/2
  Unscented Kalman Filter1/1 -> SOC2/1, SOC1/1
  SOC2/1 -> SOC/1  "k-est"
  Voltage1/1 -> Unscented Kalman Filter1/1
  Constant1/1 -> Divide1/2
  SOC1/1 -> Scope40/1, Divide1/1, Scope40/2

== system Estimations/Subsystem1/Simulink Function - Measurement Function1 ==
  Current : Inport
  Temperature (K) : Inport  Port=2
  batteryMeasurementFcn1 : TriggerPort  TriggerType=function-call  IsSimulinkFunction=on  FunctionName=batteryMeasurementFcn1  VariantControl=Variant
  Add1 : Sum  Inputs=+--
  Em Table : Lookup_n-D  BreakpointsForDimension1=SOC_LUT  BreakpointsForDimension2=Temperature_LUT  Table=Em_LUT  InternalRulePriority=Speed  RndMeth=Simplest
      settings: InputPortMap=u0,u1
  Get SOC : Selector  InputPortWidth=3  IndexOptions=Index vector (dialog)  Indices=[1]  OutputSizes=1
  Get U1 : Selector  InputPortWidth=3  IndexOptions=Index vector (dialog)  Indices=2  OutputSizes=1
  Get U2 : Selector  InputPortWidth=3  IndexOptions=Index vector (dialog)  Indices=3  OutputSizes=1
  Product : Product
  x : ArgIn  DisableCoverage=on  PortDimensions=3  ArgumentName=x1
  y : ArgOut  DisableCoverage=on  ArgumentName=y1
  wires:
  x/1 -> Get U1/1, Get U2/1, Get SOC/1
  Get SOC/1 -> Em Table/1  "SOC"
  Em Table/1 -> Add1/1
  Add1/1 -> y/1
  Temperature (K)/1 -> Em Table/2
  Get U2/1 -> Product/1
  Current/1 -> Product/2
  Product/1 -> Add1/2
  Get U1/1 -> Add1/3  "U1"

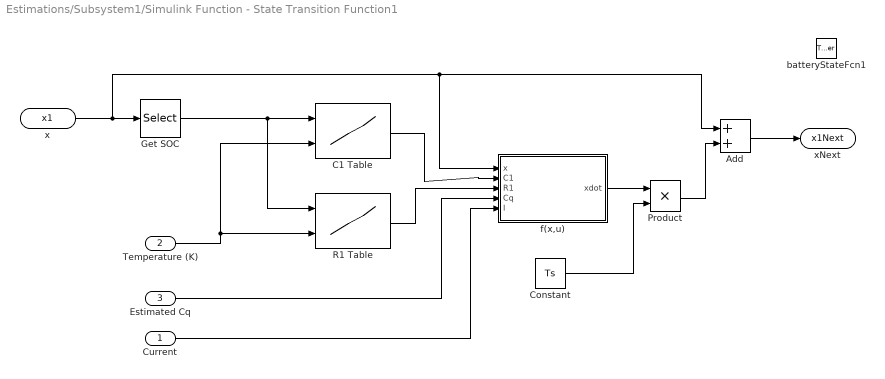
== system Estimations/Subsystem1/Simulink Function - State Transition Function1 ==
  Current : Inport
  Temperature (K) : Inport  Port=2
  Estimated Cq : Inport  Port=3
  batteryStateFcn1 : TriggerPort  TriggerType=function-call  IsSimulinkFunction=on  FunctionName=batteryStateFcn1  VariantControl=Variant
  Add : Sum
  C1 Table : Lookup_n-D  BreakpointsForDimension1=SOC_LUT  BreakpointsForDimension2=Temperature_LUT  Table=C1_LUT  InternalRulePriority=Speed  RndMeth=Simplest
      settings: InputPortMap=u0,u1
  Constant : Constant  Value=Ts
  Get SOC : Selector  InputPortWidth=3  IndexOptions=Index vector (dialog)  Indices=1  OutputSizes=1
  Product : Product
  R1 Table : Lookup_n-D  BreakpointsForDimension1=SOC_LUT  BreakpointsForDimension2=Temperature_LUT  Table=R1_LUT  InternalRulePriority=Speed  RndMeth=Simplest
      settings: InputPortMap=u0,u1
  f(x,u) : MATLAB Function  TreatAsAtomicUnit=on
  x : ArgIn  DisableCoverage=on  PortDimensions=3  ArgumentName=x1
  xNext : ArgOut  DisableCoverage=on  PortDimensions=3  ArgumentName=x1Next
  wires:
  x/1 -> f(x,u)/1(x), Add/1, Get SOC/1
  Add/1 -> xNext/1
  Temperature (K)/1 -> R1 Table/2, C1 Table/2
  Get SOC/1 -> R1 Table/1, C1 Table/1
  C1 Table/1 -> f(x,u)/2(C1)
  R1 Table/1 -> f(x,u)/3(R1)
  Current/1 -> f(x,u)/5(I)
  Constant/1 -> Product/2
  f(x,u)/1(xdot) -> Product/1
  Product/1 -> Add/2
  Estimated Cq/1 -> f(x,u)/4(Cq)

== system Estimations/Subsystem2/Simulink Function - Measurement Function2 ==
  Current : Inport
  Temperature (K) : Inport  Port=2
  batteryMeasurementFcn2 : TriggerPort  TriggerType=function-call  IsSimulinkFunction=on  FunctionName=batteryMeasurementFcn2  VariantControl=Variant
  Add1 : Sum  Inputs=+--
  Em Table : Lookup_n-D  BreakpointsForDimension1=SOC_LUT  BreakpointsForDimension2=Temperature_LUT  Table=Em_LUT  InternalRulePriority=Speed  RndMeth=Simplest
      settings: InputPortMap=u0,u1
  Get SOC : Selector  InputPortWidth=3  IndexOptions=Index vector (dialog)  Indices=[1]  OutputSizes=1
  Get U1 : Selector  InputPortWidth=3  IndexOptions=Index vector (dialog)  Indices=2  OutputSizes=1
  Get U2 : Selector  InputPortWidth=3  IndexOptions=Index vector (dialog)  Indices=3  OutputSizes=1
  Product : Product
  x1 : ArgIn  DisableCoverage=on  PortDimensions=3  ArgumentName=x1
  y1 : ArgOut  DisableCoverage=on  ArgumentName=y1
  wires:
  Get U1/1 -> Add1/3  "U1"
  Product/1 -> Add1/2
  Current/1 -> Product/2
  Get U2/1 -> Product/1
  Temperature (K)/1 -> Em Table/2
  Add1/1 -> y1/1
  Em Table/1 -> Add1/1
  Get SOC/1 -> Em Table/1  "SOC"
  x1/1 -> Get SOC/1, Get U2/1, Get U1/1

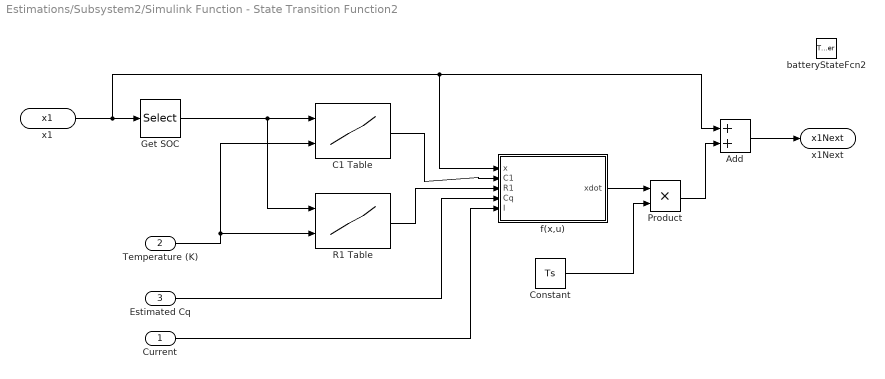
== system Estimations/Subsystem2/Simulink Function - State Transition Function2 ==
  Current : Inport
  Temperature (K) : Inport  Port=2
  Estimated Cq : Inport  Port=3
  batteryStateFcn2 : TriggerPort  TriggerType=function-call  IsSimulinkFunction=on  FunctionName=batteryStateFcn2  VariantControl=Variant
  Add : Sum
  C1 Table : Lookup_n-D  BreakpointsForDimension1=SOC_LUT  BreakpointsForDimension2=Temperature_LUT  Table=C1_LUT  InternalRulePriority=Speed  RndMeth=Simplest
      settings: InputPortMap=u0,u1
  Constant : Constant  Value=Ts
  Get SOC : Selector  InputPortWidth=3  IndexOptions=Index vector (dialog)  Indices=1  OutputSizes=1
  Product : Product
  R1 Table : Lookup_n-D  BreakpointsForDimension1=SOC_LUT  BreakpointsForDimension2=Temperature_LUT  Table=R1_LUT  InternalRulePriority=Speed  RndMeth=Simplest
      settings: InputPortMap=u0,u1
  f(x,u) : MATLAB Function  TreatAsAtomicUnit=on
  x1 : ArgIn  DisableCoverage=on  PortDimensions=3  ArgumentName=x1
  x1Next : ArgOut  DisableCoverage=on  PortDimensions=3  ArgumentName=x1Next
  wires:
  Estimated Cq/1 -> f(x,u)/4(Cq)
  Product/1 -> Add/2
  f(x,u)/1(xdot) -> Product/1
  Constant/1 -> Product/2
  Current/1 -> f(x,u)/5(I)
  R1 Table/1 -> f(x,u)/3(R1)
  C1 Table/1 -> f(x,u)/2(C1)
  Get SOC/1 -> C1 Table/1, R1 Table/1
  Temperature (K)/1 -> C1 Table/2, R1 Table/2
  Add/1 -> x1Next/1
  x1/1 -> Get SOC/1, Add/1, f(x,u)/1(x)

== system Estimations/Subsystem3/Simulink Function - Measurement Function1 ==
  Current : Inport
  Temperature (K) : Inport  Port=2
  batteryMeasurementFcn3 : TriggerPort  TriggerType=function-call  IsSimulinkFunction=on  FunctionName=batteryMeasurementFcn3  VariantControl=Variant
  Add1 : Sum  Inputs=+--
  Em Table : Lookup_n-D  BreakpointsForDimension1=SOC_LUT  BreakpointsForDimension2=Temperature_LUT  Table=Em_LUT  InternalRulePriority=Speed  RndMeth=Simplest
      settings: InputPortMap=u0,u1
  Get SOC : Selector  InputPortWidth=3  IndexOptions=Index vector (dialog)  Indices=[1]  OutputSizes=1
  Get U1 : Selector  InputPortWidth=3  IndexOptions=Index vector (dialog)  Indices=2  OutputSizes=1
  Get U2 : Selector  InputPortWidth=3  IndexOptions=Index vector (dialog)  Indices=3  OutputSizes=1
  Product : Product
  x1 : ArgIn  DisableCoverage=on  PortDimensions=3  ArgumentName=x1
  y1 : ArgOut  DisableCoverage=on  ArgumentName=y1
  wires:
  x1/1 -> Get U1/1, Get U2/1, Get SOC/1
  Get SOC/1 -> Em Table/1  "SOC"
  Em Table/1 -> Add1/1
  Add1/1 -> y1/1
  Temperature (K)/1 -> Em Table/2
  Get U2/1 -> Product/1
  Current/1 -> Product/2
  Product/1 -> Add1/2
  Get U1/1 -> Add1/3  "U1"

== system Estimations/Subsystem3/Simulink Function - State Transition Function1 ==
  Current : Inport
  Temperature (K) : Inport  Port=2
  Estimated Cq : Inport  Port=3
  batteryStateFcn3 : TriggerPort  TriggerType=function-call  IsSimulinkFunction=on  FunctionName=batteryStateFcn3  VariantControl=Variant
  Add : Sum
  C1 Table : Lookup_n-D  BreakpointsForDimension1=SOC_LUT  BreakpointsForDimension2=Temperature_LUT  Table=C1_LUT  InternalRulePriority=Speed  RndMeth=Simplest
      settings: InputPortMap=u0,u1
  Constant : Constant  Value=Ts
  Get SOC : Selector  InputPortWidth=3  IndexOptions=Index vector (dialog)  Indices=1  OutputSizes=1
  Product : Product
  R1 Table : Lookup_n-D  BreakpointsForDimension1=SOC_LUT  BreakpointsForDimension2=Temperature_LUT  Table=R1_LUT  InternalRulePriority=Speed  RndMeth=Simplest
      settings: InputPortMap=u0,u1
  f(x,u) : MATLAB Function  TreatAsAtomicUnit=on
  x1 : ArgIn  DisableCoverage=on  PortDimensions=3  ArgumentName=x1
  x1Next : ArgOut  DisableCoverage=on  PortDimensions=3  ArgumentName=x1Next
  wires:
  x1/1 -> f(x,u)/1(x), Add/1, Get SOC/1
  Add/1 -> x1Next/1
  Temperature (K)/1 -> R1 Table/2, C1 Table/2
  Get SOC/1 -> R1 Table/1, C1 Table/1
  C1 Table/1 -> f(x,u)/2(C1)
  R1 Table/1 -> f(x,u)/3(R1)
  Current/1 -> f(x,u)/5(I)
  Constant/1 -> Product/2
  f(x,u)/1(xdot) -> Product/1
  Product/1 -> Add/2
  Estimated Cq/1 -> f(x,u)/4(Cq)

== system Estimations/Subsystem4/Simulink Function - Measurement Function1 ==
  Current : Inport
  Temperature (K) : Inport  Port=2
  batteryMeasurementFcn4 : TriggerPort  TriggerType=function-call  IsSimulinkFunction=on  FunctionName=batteryMeasurementFcn4  VariantControl=Variant
  Add1 : Sum  Inputs=+--
  Em Table : Lookup_n-D  BreakpointsForDimension1=SOC_LUT  BreakpointsForDimension2=Temperature_LUT  Table=Em_LUT  InternalRulePriority=Speed  RndMeth=Simplest
      settings: InputPortMap=u0,u1
  Get SOC : Selector  InputPortWidth=3  IndexOptions=Index vector (dialog)  Indices=[1]  OutputSizes=1
  Get U1 : Selector  InputPortWidth=3  IndexOptions=Index vector (dialog)  Indices=2  OutputSizes=1
  Get U2 : Selector  InputPortWidth=3  IndexOptions=Index vector (dialog)  Indices=3  OutputSizes=1
  Product : Product
  x1 : ArgIn  DisableCoverage=on  PortDimensions=3  ArgumentName=x1
  y1 : ArgOut  DisableCoverage=on  ArgumentName=y1
  wires:
  Get U1/1 -> Add1/3  "U1"
  Product/1 -> Add1/2
  Current/1 -> Product/2
  Get U2/1 -> Product/1
  Temperature (K)/1 -> Em Table/2
  Add1/1 -> y1/1
  Em Table/1 -> Add1/1
  Get SOC/1 -> Em Table/1  "SOC"
  x1/1 -> Get SOC/1, Get U2/1, Get U1/1

== system Estimations/Subsystem4/Simulink Function - State Transition Function1 ==
  Current : Inport
  Temperature (K) : Inport  Port=2
  Estimated Cq : Inport  Port=3
  batteryStateFcn4 : TriggerPort  TriggerType=function-call  IsSimulinkFunction=on  FunctionName=batteryStateFcn4  VariantControl=Variant
  Add : Sum
  C1 Table : Lookup_n-D  BreakpointsForDimension1=SOC_LUT  BreakpointsForDimension2=Temperature_LUT  Table=C1_LUT  InternalRulePriority=Speed  RndMeth=Simplest
      settings: InputPortMap=u0,u1
  Constant : Constant  Value=Ts
  Get SOC : Selector  InputPortWidth=3  IndexOptions=Index vector (dialog)  Indices=1  OutputSizes=1
  Product : Product
  R1 Table : Lookup_n-D  BreakpointsForDimension1=SOC_LUT  BreakpointsForDimension2=Temperature_LUT  Table=R1_LUT  InternalRulePriority=Speed  RndMeth=Simplest
      settings: InputPortMap=u0,u1
  f(x,u) : MATLAB Function  TreatAsAtomicUnit=on
  x1 : ArgIn  DisableCoverage=on  PortDimensions=3  ArgumentName=x1
  x1Next : ArgOut  DisableCoverage=on  PortDimensions=3  ArgumentName=x1Next
  wires:
  Estimated Cq/1 -> f(x,u)/4(Cq)
  Product/1 -> Add/2
  f(x,u)/1(xdot) -> Product/1
  Constant/1 -> Product/2
  Current/1 -> f(x,u)/5(I)
  R1 Table/1 -> f(x,u)/3(R1)
  C1 Table/1 -> f(x,u)/2(C1)
  Get SOC/1 -> C1 Table/1, R1 Table/1
  Temperature (K)/1 -> C1 Table/2, R1 Table/2
  Add/1 -> x1Next/1
  x1/1 -> Get SOC/1, Add/1, f(x,u)/1(x)

== system Estimations/Subsystem5/Simulink Function - Measurement Function1 ==
  Current : Inport
  Temperature (K) : Inport  Port=2
  batteryMeasurementFcn5 : TriggerPort  TriggerType=function-call  IsSimulinkFunction=on  FunctionName=batteryMeasurementFcn5  VariantControl=Variant
  Add1 : Sum  Inputs=+--
  Em Table : Lookup_n-D  BreakpointsForDimension1=SOC_LUT  BreakpointsForDimension2=Temperature_LUT  Table=Em_LUT  InternalRulePriority=Speed  RndMeth=Simplest
      settings: InputPortMap=u0,u1
  Get SOC : Selector  InputPortWidth=3  IndexOptions=Index vector (dialog)  Indices=[1]  OutputSizes=1
  Get U1 : Selector  InputPortWidth=3  IndexOptions=Index vector (dialog)  Indices=2  OutputSizes=1
  Get U2 : Selector  InputPortWidth=3  IndexOptions=Index vector (dialog)  Indices=3  OutputSizes=1
  Product : Product
  x1 : ArgIn  DisableCoverage=on  PortDimensions=3  ArgumentName=x1
  y1 : ArgOut  DisableCoverage=on  ArgumentName=y1
  wires:
  x1/1 -> Get U1/1, Get U2/1, Get SOC/1
  Get SOC/1 -> Em Table/1  "SOC"
  Em Table/1 -> Add1/1
  Add1/1 -> y1/1
  Temperature (K)/1 -> Em Table/2
  Get U2/1 -> Product/1
  Current/1 -> Product/2
  Product/1 -> Add1/2
  Get U1/1 -> Add1/3  "U1"

== system Estimations/Subsystem5/Simulink Function - State Transition Function1 ==
  Current : Inport
  Temperature (K) : Inport  Port=2
  Estimated Cq : Inport  Port=3
  batteryStateFcn5 : TriggerPort  TriggerType=function-call  IsSimulinkFunction=on  FunctionName=batteryStateFcn5  VariantControl=Variant
  Add : Sum
  C1 Table : Lookup_n-D  BreakpointsForDimension1=SOC_LUT  BreakpointsForDimension2=Temperature_LUT  Table=C1_LUT  InternalRulePriority=Speed  RndMeth=Simplest
      settings: InputPortMap=u0,u1
  Constant : Constant  Value=Ts
  Get SOC : Selector  InputPortWidth=3  IndexOptions=Index vector (dialog)  Indices=1  OutputSizes=1
  Product : Product
  R1 Table : Lookup_n-D  BreakpointsForDimension1=SOC_LUT  BreakpointsForDimension2=Temperature_LUT  Table=R1_LUT  InternalRulePriority=Speed  RndMeth=Simplest
      settings: InputPortMap=u0,u1
  f(x,u) : MATLAB Function  TreatAsAtomicUnit=on
  x1 : ArgIn  DisableCoverage=on  PortDimensions=3  ArgumentName=x1
  x1Next : ArgOut  DisableCoverage=on  PortDimensions=3  ArgumentName=x1Next
  wires:
  x1/1 -> f(x,u)/1(x), Add/1, Get SOC/1
  Add/1 -> x1Next/1
  Temperature (K)/1 -> R1 Table/2, C1 Table/2
  Get SOC/1 -> R1 Table/1, C1 Table/1
  C1 Table/1 -> f(x,u)/2(C1)
  R1 Table/1 -> f(x,u)/3(R1)
  Current/1 -> f(x,u)/5(I)
  Constant/1 -> Product/2
  f(x,u)/1(xdot) -> Product/1
  Product/1 -> Add/2
  Estimated Cq/1 -> f(x,u)/4(Cq)

== system Estimations/Subsystem6/Simulink Function - Measurement Function1 ==
  Current : Inport
  Temperature (K) : Inport  Port=2
  batteryMeasurementFcn6 : TriggerPort  TriggerType=function-call  IsSimulinkFunction=on  FunctionName=batteryMeasurementFcn6  VariantControl=Variant
  Add1 : Sum  Inputs=+--
  Em Table : Lookup_n-D  BreakpointsForDimension1=SOC_LUT  BreakpointsForDimension2=Temperature_LUT  Table=Em_LUT  InternalRulePriority=Speed  RndMeth=Simplest
      settings: InputPortMap=u0,u1
  Get SOC : Selector  InputPortWidth=3  IndexOptions=Index vector (dialog)  Indices=[1]  OutputSizes=1
  Get U1 : Selector  InputPortWidth=3  IndexOptions=Index vector (dialog)  Indices=2  OutputSizes=1
  Get U2 : Selector  InputPortWidth=3  IndexOptions=Index vector (dialog)  Indices=3  OutputSizes=1
  Product : Product
  x1 : ArgIn  DisableCoverage=on  PortDimensions=3  ArgumentName=x1
  y1 : ArgOut  DisableCoverage=on  ArgumentName=y1
  wires:
  Get U1/1 -> Add1/3  "U1"
  Product/1 -> Add1/2
  Current/1 -> Product/2
  Get U2/1 -> Product/1
  Temperature (K)/1 -> Em Table/2
  Add1/1 -> y1/1
  Em Table/1 -> Add1/1
  Get SOC/1 -> Em Table/1  "SOC"
  x1/1 -> Get SOC/1, Get U2/1, Get U1/1
